simulink subsystem "plantDynamics2019"  (R2019b)
settings: Solver=VariableStepAuto  StartTime=0.0  StopTime=10.0  RelTol=1e-3
InitFcn:
  | parameters
values from neighbouring files (symbols this model uses):
  A = [-1/(R_is*C_s) 1/(R_is*C_s) 0 0 ... (first row only)    [SSModel.m]
  B = [0; 0; Phi_h/C_h; 0]    [SSModel.m]
  C = [1 0 0 0]    [SSModel.m]
  E = [0 0; 0 A_w/C_i; 0 0; 1/(R_ea*C_e) A_e/C_e]    [SSModel.m]
  x_0 = [20; 20; 20; 20]    [parameters.m]
settings Model: Creator=micha  LastModifiedBy=micha

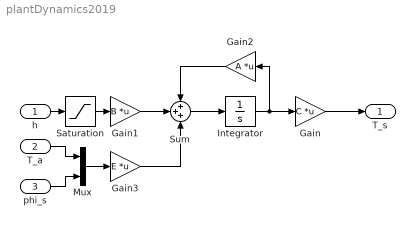
== system plantDynamics2019 ==
  h : Inport
  T_a : Inport  Port=2
  phi_s : Inport  Port=3
  Gain : Gain  InitFcn=parameters  Gain=C  Multiplication=Matrix(K*u)
  Gain1 : Gain  Gain=B  Multiplication=Matrix(K*u)
  Gain2 : Gain  Gain=A  Multiplication=Matrix(K*u)
  Gain3 : Gain  Gain=E  Multiplication=Matrix(K*u)
  Integrator : Integrator  InitialCondition=x_0
  Mux : Mux  Inputs=2
  Saturation : Saturate  UpperLimit=1  LowerLimit=0
  Sum : Sum  Inputs=+++
  T_s : Outport
  wires:
  Integrator/1 -> Gain2/1, Gain/1
  Sum/1 -> Integrator/1
  Gain1/1 -> Sum/2
  Gain2/1 -> Sum/1
  Gain3/1 -> Sum/3
  Mux/1 -> Gain3/1
  Gain/1 -> T_s/1
  phi_s/1 -> Mux/2
  h/1 -> Saturation/1
  Saturation/1 -> Gain1/1
  T_a/1 -> Mux/1
